simulink model "Task_01_Sim"  (R2024a)
settings: Solver=VariableStepAuto  StartTime=0.0  StopTime=40.0  RelTol=1e-3
settings Model: Creator=PMYLS  LastModifiedBy=PMYLS

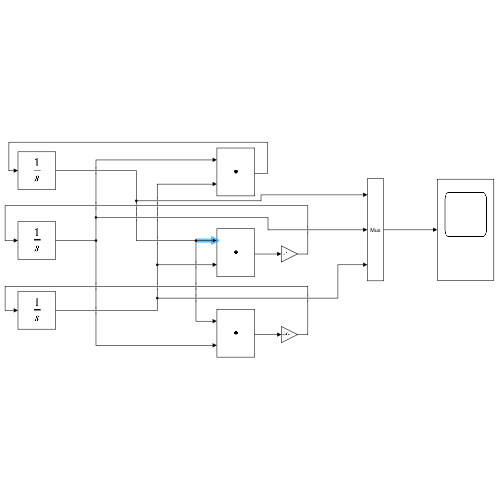
[thumbnail: Simulink's stored preview of the top-level diagram]
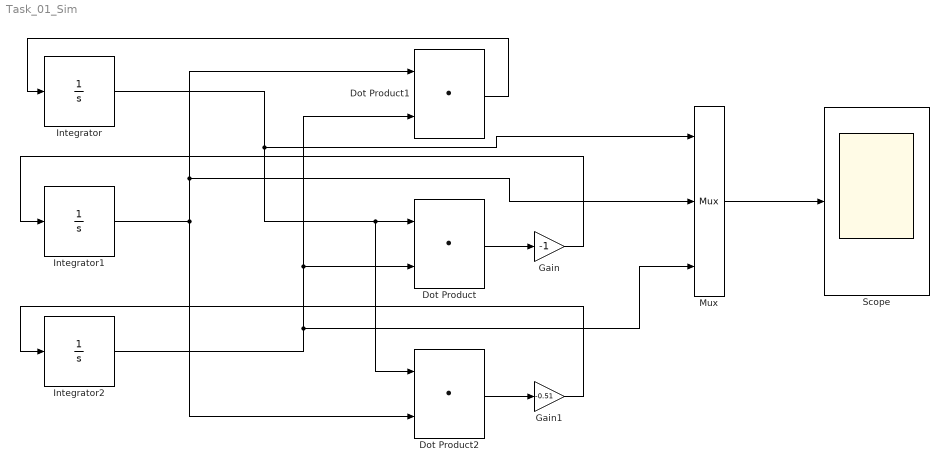
== system Task_01_Sim ==
  Dot Product : DotProduct  OutDataTypeStr=Inherit: Inherit via internal rule
  Dot Product1 : DotProduct  OutDataTypeStr=Inherit: Inherit via internal rule
  Dot Product2 : DotProduct  OutDataTypeStr=Inherit: Inherit via internal rule
  Gain : Gain  Gain=-1
  Gain1 : Gain  Gain=-0.51
  Integrator : Integrator
  Integrator1 : Integrator  InitialCondition=1
  Integrator2 : Integrator  InitialCondition=1
  Mux : Mux  Inputs=3
  Scope : Scope
  wires:
  Mux/1 -> Scope/1
  Dot Product1/1 -> Integrator/1
  Dot Product/1 -> Gain/1
  Gain/1 -> Integrator1/1
  Dot Product2/1 -> Gain1/1
  Gain1/1 -> Integrator2/1
  Integrator/1 -> Mux/1, Dot Product2/1, Dot Product/1
  Integrator2/1 -> Mux/3, Dot Product/2, Dot Product1/2
  Integrator1/1 -> Mux/2, Dot Product1/1, Dot Product2/2
